simulink model "rotations_test"  (R2018b)
settings: Solver=VariableStepAuto  StartTime=0.0  StopTime=0  RelTol=1e-3
values from neighbouring files (symbols this model uses):
  jdut1 = 2453101.82740678    (= 2453101.82741)    [DCM_UnitTest_MATLAB.m]
  ttt = 0.0426236319    [DCM_UnitTest_MATLAB.m]
libraries: rotations_Lib x1
settings Model: Creator=IvanMachuca  LastModifiedBy=IvanMachuca

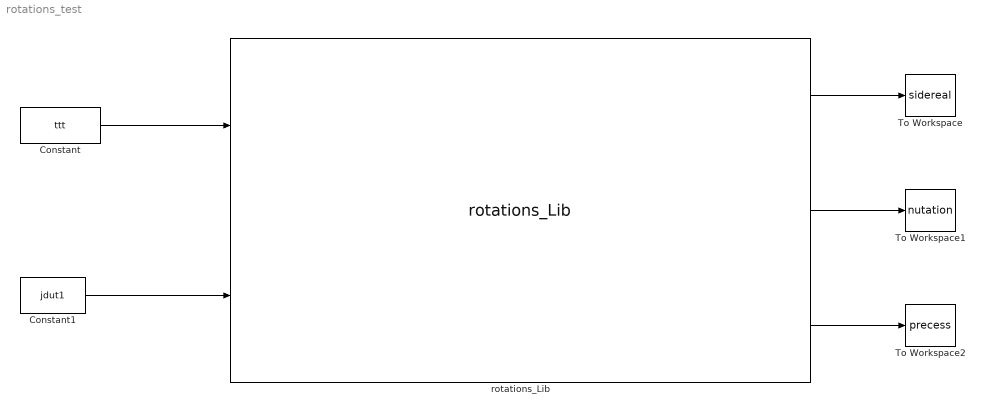
== system rotations_test ==
  Constant : Constant  Value=ttt
  Constant1 : Constant  Value=jdut1
  To Workspace : ToWorkspace  VariableName=sidereal  SampleTime=-1
      settings: Save2DSignal=2-D array (concatenate along first dimension)
  To Workspace1 : ToWorkspace  VariableName=nutation  SampleTime=-1
      settings: Save2DSignal=2-D array (concatenate along first dimension)
  To Workspace2 : ToWorkspace  VariableName=precess  SampleTime=-1
      settings: Save2DSignal=2-D array (concatenate along first dimension)
  "rotations_Lib " : rotations_Lib/rotations_Lib    SystemSampleTime=-1
  wires:
  "rotations_Lib "/1 -> To Workspace/1
  "rotations_Lib "/2 -> To Workspace1/1
  "rotations_Lib "/3 -> To Workspace2/1
  Constant/1 -> "rotations_Lib "/1
  Constant1/1 -> "rotations_Lib "/2
